simulink model "homework2pro"  (R2018a)
settings: Solver=VariableStepAuto  StartTime=0.0  StopTime=30.0  RelTol=1e-5
undefined symbols (not defined in the file): y0, y1, y2, y3
settings Model: Creator=dell  LastModifiedBy=dell

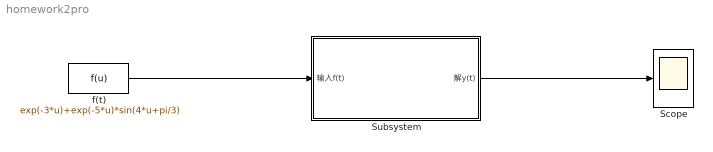
== system homework2pro ==
  Scope : Scope
      settings: StartFcn=open_system(gcbh);
  Subsystem : Subsystem  mask(Sove ODE4){Parameter4=3, Parameter1=3, Parameter2=4, Parameter3=5}
      mask prompts: Parameter4 "a3"; Parameter1 "a2"; Parameter2 "a1"; Parameter3 "a0"
      mask help:
      | 求解y''''+a3y'''+a2y''+a1y'+a0y=f(t)形式的微分方程
      | 初始条件y'''(0)=y3, y''(0)=y2, y'(0)=y1, y(0)=y0
  f(t) : Fcn  Expr=exp(-3*u)+exp(-5*u)*sin(4*u+pi/3)
  wires:
  f(t)/1 -> Subsystem/1(输入f(t))
  Subsystem/1(解y(t)) -> Scope/1

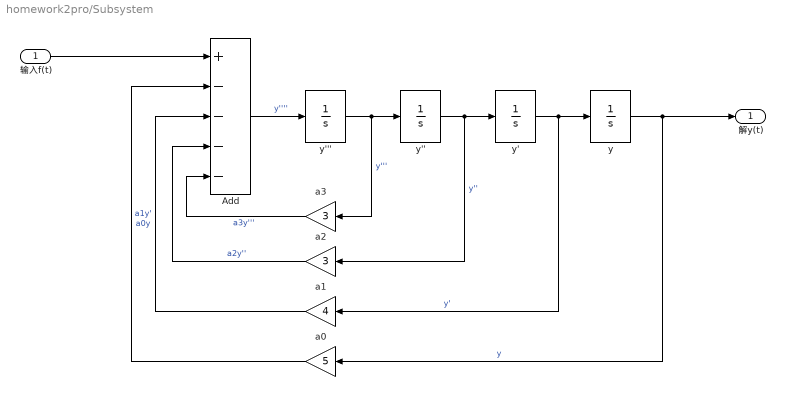
== system homework2pro/Subsystem ==
  输入f(t) : Inport
  Add : Sum  Inputs=+----
  a0 : Gain  Gain=5
  a1 : Gain  Gain=4
  a2 : Gain  Gain=3
  a3 : Gain  Gain=3
  y : Integrator  InitialCondition=y0
  y' : Integrator  InitialCondition=y1
  y'' : Integrator  InitialCondition=y2
  y''' : Integrator  InitialCondition=y3
  解y(t) : Outport
  wires:
  a0/1 -> Add/2  "a0y"
  a1/1 -> Add/3  "a1y'"
  y'''/1 -> a3/1, y''/1  "y'''"
  y/1 -> 解y(t)/1, a0/1  "y"
  y'/1 -> a1/1, y/1  "y'"
  Add/1 -> y'''/1  "y''''"
  y''/1 -> a2/1, y'/1  "y''"
  a2/1 -> Add/4  "a2y''"
  a3/1 -> Add/5  "a3y'''"
  输入f(t)/1 -> Add/1
